simulink model "IEEE14_case"  (R2024b)
settings: Solver=FixedStepAuto  StartTime=0  StopTime=2  FixedStep=1e-7  RelTol=1e-3
values from neighbouring files (symbols this model uses):
  GFL_15_Bva = 0.009    [IEEE14_parameters.m]
  GFL_15_C_bus_pu = 7.179419    [IEEE14_parameters.m]
  GFL_15_f0 = 60    [IEEE14_parameters.m]
  GFL_15_I_id = 691.26967    [IEEE14_parameters.m]
  GFL_15_I_iq = 691.26967    [IEEE14_parameters.m]
  GFL_15_I_od = 45.2207    [IEEE14_parameters.m]
  GFL_15_I_oq = 45.2207    [IEEE14_parameters.m]
  GFL_15_I_pll = 0.78    [IEEE14_parameters.m]
  GFL_15_Kdi = 0.09    [IEEE14_parameters.m]
  GFL_15_Kdo = 0.9    [IEEE14_parameters.m]
  GFL_15_Kqi = 0.09    [IEEE14_parameters.m]
  GFL_15_Kqo = 0.9    [IEEE14_parameters.m]
  GFL_15_Lg_pu = 0.631447    [IEEE14_parameters.m]
  GFL_15_mode = 1    [IEEE14_parameters.m]
  GFL_15_P_id = 3.7166    [IEEE14_parameters.m]
  GFL_15_P_iq = 3.7166    [IEEE14_parameters.m]
  GFL_15_P_od = 0.4798    [IEEE14_parameters.m]
  GFL_15_P_oq = 0.4798    [IEEE14_parameters.m]
  GFL_15_P_pll = 290.42    [IEEE14_parameters.m]
  GFL_15_Qe_ref = 0.2    [IEEE14_parameters.m]
  GFL_15_Rg_pu = 0.024016    [IEEE14_parameters.m]
  GFL_15_Sbase = 1.000000e+4    (= 10000)    [IEEE14_parameters.m]
  GFL_15_Tdi = 0.01    [IEEE14_parameters.m]
  GFL_15_Tdo = 0.2    [IEEE14_parameters.m]
  GFL_15_Tqi = 0.01    [IEEE14_parameters.m]
  GFL_15_Tqo = 0.2    [IEEE14_parameters.m]
  GFL_15_Vbase = 380    [IEEE14_parameters.m]
  GFL_15_Vdc_ref = 1.011475    [IEEE14_parameters.m]
  GFL_15_Vdcbase = 700    [IEEE14_parameters.m]
  GFL_15_vq_ref = 0    [IEEE14_parameters.m]
  GFL_16_Bva = 0.002    [IEEE14_parameters.m]
  GFL_16_C_bus_pu = 7.179419    [IEEE14_parameters.m]
  GFL_16_f0 = 60    [IEEE14_parameters.m]
  GFL_16_I_id = 691.26967    [IEEE14_parameters.m]
  GFL_16_I_iq = 691.26967    [IEEE14_parameters.m]
  GFL_16_I_od = 45.2207    [IEEE14_parameters.m]
  GFL_16_I_oq = 45.2207    [IEEE14_parameters.m]
  GFL_16_I_pll = 0.78    [IEEE14_parameters.m]
  GFL_16_Kdi = 0.05    [IEEE14_parameters.m]
  GFL_16_Kdo = 0.5    [IEEE14_parameters.m]
  GFL_16_Kqi = 0.05    [IEEE14_parameters.m]
  GFL_16_Kqo = 0.5    [IEEE14_parameters.m]
  GFL_16_Lg_pu = 0.631447    [IEEE14_parameters.m]
  GFL_16_mode = 1    [IEEE14_parameters.m]
  GFL_16_P_id = 3.7166    [IEEE14_parameters.m]
  GFL_16_P_iq = 3.7166    [IEEE14_parameters.m]
  GFL_16_P_od = 0.4798    [IEEE14_parameters.m]
  GFL_16_P_oq = 0.4798    [IEEE14_parameters.m]
  GFL_16_P_pll = 290.42    [IEEE14_parameters.m]
  GFL_16_Qe_ref = 0.2    [IEEE14_parameters.m]
  GFL_16_Rg_pu = 0.024016    [IEEE14_parameters.m]
  GFL_16_Sbase = 1.000000e+4    (= 10000)    [IEEE14_parameters.m]
  GFL_16_Tdi = 0.01    [IEEE14_parameters.m]
  GFL_16_Tdo = 0.2    [IEEE14_parameters.m]
  GFL_16_Tqi = 0.01    [IEEE14_parameters.m]
  GFL_16_Tqo = 0.2    [IEEE14_parameters.m]
  GFL_16_Vbase = 380    [IEEE14_parameters.m]
  GFL_16_Vdc_ref = 1.01144    [IEEE14_parameters.m]
  GFL_16_Vdcbase = 700    [IEEE14_parameters.m]
  GFL_16_vq_ref = 0    [IEEE14_parameters.m]
  GFL_17_Bva = 0.002    [IEEE14_parameters.m]
  GFL_17_C_bus_pu = 7.179419    [IEEE14_parameters.m]
  GFL_17_f0 = 60    [IEEE14_parameters.m]
  GFL_17_I_id = 691.26967    [IEEE14_parameters.m]
  GFL_17_I_iq = 691.26967    [IEEE14_parameters.m]
  GFL_17_I_od = 45.2207    [IEEE14_parameters.m]
  GFL_17_I_oq = 45.2207    [IEEE14_parameters.m]
  GFL_17_I_pll = 0.78    [IEEE14_parameters.m]
  GFL_17_Kdi = 0.05    [IEEE14_parameters.m]
  GFL_17_Kdo = 0.5    [IEEE14_parameters.m]
  GFL_17_Kqi = 0.05    [IEEE14_parameters.m]
  GFL_17_Kqo = 0.5    [IEEE14_parameters.m]
  GFL_17_Lg_pu = 0.631447    [IEEE14_parameters.m]
  GFL_17_mode = 1    [IEEE14_parameters.m]
  GFL_17_P_id = 3.7166    [IEEE14_parameters.m]
  GFL_17_P_iq = 3.7166    [IEEE14_parameters.m]
  GFL_17_P_od = 0.4798    [IEEE14_parameters.m]
  GFL_17_P_oq = 0.4798    [IEEE14_parameters.m]
  GFL_17_P_pll = 290.42    [IEEE14_parameters.m]
  GFL_17_Qe_ref = 0.2    [IEEE14_parameters.m]
  GFL_17_Rg_pu = 0.024016    [IEEE14_parameters.m]
  GFL_17_Sbase = 1.000000e+4    (= 10000)    [IEEE14_parameters.m]
  GFL_17_Tdi = 0.01    [IEEE14_parameters.m]
  GFL_17_Tdo = 0.2    [IEEE14_parameters.m]
  GFL_17_Tqi = 0.01    [IEEE14_parameters.m]
  GFL_17_Tqo = 0.2    [IEEE14_parameters.m]
  GFL_17_Vbase = 380    [IEEE14_parameters.m]
  GFL_17_Vdc_ref = 1.011632    [IEEE14_parameters.m]
  GFL_17_Vdcbase = 700    [IEEE14_parameters.m]
  GFL_17_vq_ref = 0    [IEEE14_parameters.m]
  GFL_18_Bva = 0.002    [IEEE14_parameters.m]
  GFL_18_C_bus_pu = 7.179419    [IEEE14_parameters.m]
  GFL_18_f0 = 60    [IEEE14_parameters.m]
  GFL_18_I_id = 691.26967    [IEEE14_parameters.m]
  GFL_18_I_iq = 691.26967    [IEEE14_parameters.m]
  GFL_18_I_od = 45.2207    [IEEE14_parameters.m]
  GFL_18_I_oq = 45.2207    [IEEE14_parameters.m]
  GFL_18_I_pll = 0.78    [IEEE14_parameters.m]
  GFL_18_Kdi = 0.05    [IEEE14_parameters.m]
  GFL_18_Kdo = 0.5    [IEEE14_parameters.m]
  GFL_18_Kqi = 0.05    [IEEE14_parameters.m]
  GFL_18_Kqo = 0.5    [IEEE14_parameters.m]
  GFL_18_Lg_pu = 0.631447    [IEEE14_parameters.m]
  GFL_18_mode = 1    [IEEE14_parameters.m]
  GFL_18_P_id = 3.7166    [IEEE14_parameters.m]
  GFL_18_P_iq = 3.7166    [IEEE14_parameters.m]
  GFL_18_P_od = 0.4798    [IEEE14_parameters.m]
  GFL_18_P_oq = 0.4798    [IEEE14_parameters.m]
  GFL_18_P_pll = 290.42    [IEEE14_parameters.m]
  GFL_18_Qe_ref = 0.2    [IEEE14_parameters.m]
  GFL_18_Rg_pu = 0.024016    [IEEE14_parameters.m]
  GFL_18_Sbase = 1.000000e+4    (= 10000)    [IEEE14_parameters.m]
  GFL_18_Tdi = 0.01    [IEEE14_parameters.m]
  GFL_18_Tdo = 0.2    [IEEE14_parameters.m]
  GFL_18_Tqi = 0.01    [IEEE14_parameters.m]
  GFL_18_Tqo = 0.2    [IEEE14_parameters.m]
  GFL_18_Vbase = 380    [IEEE14_parameters.m]
  GFL_18_Vdc_ref = 1.011572    [IEEE14_parameters.m]
  GFL_18_Vdcbase = 700    [IEEE14_parameters.m]
  GFL_18_vq_ref = 0    [IEEE14_parameters.m]
  ... (+180 more)
(part 21 of 25)

== system IEEE14_case/SG_D_3/i_q_SG_D_3_block ==
  note: i_q_SG_D_3 in case14gfl
      | $-\frac{\sin\left(\theta _{\mathrm{SG},D,3}\right)\,\left(\psi _{q,\mathrm{SG},D,3}+\frac{\psi _{\mathrm{gq},\mathrm{SG},D,3}\,\left(x_{l}-x_{\mathrm{qdd}}\right)}{x_{l}-x_{\mathrm{qd}}}+\frac{\psi _{\mathrm{kq},\mathrm{SG},D,3}\,\left(x_{\mathrm{qd}}-x_{\mathrm{qdd}}\right)}{x_{l}-x_{\mathrm{qd}}}\right)}{x_{\mathrm{qdd}}}-\frac{\cos\left(\theta _{\mathrm{SG},D,3}\right)\,\left(\frac{\psi _{\mathrm{1d},\mathrm{SG},D,3}\,\left(x_{\mathrm{dd}}-x_{\mathrm{ddd}}\right)}{x_{\mathrm{dd}}-x_{l}}-\psi _{d,\mathrm{SG},D,3}+\frac{\psi _{\mathrm{fd},\mathrm{SG},D,3}\,\left(x_{\mathrm{ddd}}-x_{l}\right)}{x_{\mathrm{dd}}-x_{l}}\right)}{x_{\mathrm{ddd}}}$
      | Automatically generated on 2025-10-09 21:32:35 .
  State_psi_gq_SG_D_3_f7c17 : Inport
  State_psi_kq_SG_D_3_3c737 : Inport  Port=2
  State_psi_q_SG_D_3_2676a : Inport  Port=3
  State_theta_SG_D_3_9134c : Inport  Port=4
  State_psi_1d_SG_D_3_20d6e : Inport  Port=5
  State_psi_d_SG_D_3_ac680 : Inport  Port=6
  State_psi_fd_SG_D_3_bfdd7 : Inport  Port=7
  State_theta_SG_D_3_28037 : Inport  Port=8
  Add_4ac66 : Sum
  Add_5b661 : Sum
  Add_73f87 : Sum
  Add_78fd5 : Sum
  Add_d5f9a : Sum
  Add_dc007 : Sum
  Constant_-1_294ca : Constant  Value=-1
  Constant_-1_37339 : Constant  Value=-1
  Constant_-1_55310 : Constant  Value=-1
  Constant_-1_9bd92 : Constant  Value=-1
  Constant_-1_c0d20 : Constant  Value=-1
  Constant_x_dd_0e9f5 : Constant  Value=x_dd
  Constant_x_dd_107ff : Constant  Value=x_dd
  Constant_x_dd_c8724 : Constant  Value=x_dd
  Constant_x_ddd_0cb6a : Constant  Value=x_ddd
  Constant_x_ddd_61310 : Constant  Value=x_ddd
  Constant_x_ddd_6486c : Constant  Value=x_ddd
  Constant_x_l_1c7d3 : Constant  Value=x_l
  Constant_x_l_2af64 : Constant  Value=x_l
  Constant_x_l_57051 : Constant  Value=x_l
  Constant_x_l_7ebbc : Constant  Value=x_l
  Constant_x_l_96cf1 : Constant  Value=x_l
  Constant_x_l_9ef0a : Constant  Value=x_l
  Constant_x_qd_2bf67 : Constant  Value=x_qd
  Constant_x_qd_2ffe8 : Constant  Value=x_qd
  Constant_x_qd_baa51 : Constant  Value=x_qd
  Constant_x_qdd_09938 : Constant  Value=x_qdd
  Constant_x_qdd_17dfa : Constant  Value=x_qdd
  Constant_x_qdd_d3279 : Constant  Value=x_qdd
  Divide_0acbf : Product  Inputs=*/
  Divide_1822e : Product  Inputs=*/
  Divide_1e6a6 : Product  Inputs=*/
  Divide_3e273 : Product  Inputs=*/
  Divide_85360 : Product  Inputs=*/
  Divide_9dfff : Product  Inputs=*/
  MathFunc_cos_15d9a : Trigonometry  Operator=cos
  MathFunc_sin_902a4 : Trigonometry
  Product_0a2eb : Product
  Product_3ac28 : Product
  Product_4e1f4 : Product
  Product_5bceb : Product
  Product_723b0 : Product
  Product_7a0a1 : Product
  Product_9fc52 : Product
  Product_a5c0c : Product
  Product_ab665 : Product
  Product_b175d : Product
  Product_d7f70 : Product
  Subtract_0cd7d : Sum  Inputs=+-
  Subtract_369cd : Sum  Inputs=+-
  Subtract_41eed : Sum  Inputs=+-
  Subtract_9b04e : Sum  Inputs=+-
  Subtract_9e824 : Sum  Inputs=+-
  Subtract_b9947 : Sum  Inputs=+-
  Subtract_c0717 : Sum  Inputs=+-
  Blockout_i_q_SG_D_3_e7589 : Outport
  wires:
  Constant_x_qdd_09938/1 -> Divide_1e6a6/2
  Constant_x_dd_0e9f5/1 -> Subtract_b9947/1
  Constant_-1_37339/1 -> Product_3ac28/1
  Constant_-1_294ca/1 -> Product_b175d/1
  Constant_x_l_9ef0a/1 -> Product_b175d/2
  Subtract_41eed/1 -> Product_d7f70/1
  Constant_x_qdd_d3279/1 -> Subtract_c0717/2
  Constant_x_qdd_17dfa/1 -> Add_5b661/2
  Product_b175d/1 -> Add_5b661/1
  Constant_x_l_7ebbc/1 -> Subtract_b9947/2
  Add_d5f9a/1 -> Divide_9dfff/2
  Constant_x_l_57051/1 -> Product_3ac28/2
  Constant_x_ddd_61310/1 -> Subtract_369cd/1
  Constant_x_qd_2ffe8/1 -> Subtract_c0717/1
  Constant_-1_c0d20/1 -> Product_7a0a1/1
  Product_9fc52/1 -> Product_5bceb/1
  Constant_x_l_2af64/1 -> Product_7a0a1/2
  Product_5bceb/1 -> Divide_1822e/1
  State_psi_gq_SG_D_3_f7c17/1 -> Product_0a2eb/1
  Add_5b661/1 -> Product_0a2eb/2
  Subtract_b9947/1 -> Divide_1822e/2
  Product_3ac28/1 -> Add_d5f9a/1
  Divide_3e273/1 -> Add_4ac66/2
  Constant_x_qd_2bf67/1 -> Add_d5f9a/2
  State_psi_fd_SG_D_3_bfdd7/1 -> Product_4e1f4/1
  State_psi_kq_SG_D_3_3c737/1 -> Product_ab665/1
  Subtract_369cd/1 -> Product_4e1f4/2
  Subtract_c0717/1 -> Product_ab665/2
  Product_7a0a1/1 -> Add_73f87/1
  Constant_x_qd_baa51/1 -> Add_73f87/2
  Constant_x_l_96cf1/1 -> Subtract_369cd/2
  Constant_-1_55310/1 -> Product_9fc52/1
  State_psi_1d_SG_D_3_20d6e/1 -> Product_9fc52/2
  Constant_x_dd_c8724/1 -> Subtract_9b04e/1
  Constant_-1_9bd92/1 -> Product_723b0/1
  Constant_x_ddd_0cb6a/1 -> Subtract_9b04e/2
  Add_dc007/1 -> Product_723b0/2
  Product_0a2eb/1 -> Divide_9dfff/1
  Product_4e1f4/1 -> Divide_85360/1
  Product_ab665/1 -> Divide_0acbf/1
  Subtract_0cd7d/1 -> Divide_85360/2
  Add_73f87/1 -> Divide_0acbf/2
  Constant_x_ddd_6486c/1 -> Divide_3e273/2
  Subtract_9b04e/1 -> Product_5bceb/2
  Divide_9dfff/1 -> Subtract_9e824/1
  Divide_85360/1 -> Subtract_41eed/2
  Divide_0acbf/1 -> Subtract_9e824/2
  Constant_x_dd_107ff/1 -> Subtract_0cd7d/1
  Constant_x_l_1c7d3/1 -> Subtract_0cd7d/2
  Subtract_9e824/1 -> Add_dc007/1
  State_psi_q_SG_D_3_2676a/1 -> Add_dc007/2
  Divide_1822e/1 -> Add_78fd5/1
  MathFunc_sin_902a4/1 -> Product_a5c0c/2
  Product_723b0/1 -> Product_a5c0c/1
  State_psi_d_SG_D_3_ac680/1 -> Add_78fd5/2
  State_theta_SG_D_3_9134c/1 -> MathFunc_sin_902a4/1
  Add_78fd5/1 -> Subtract_41eed/1
  State_theta_SG_D_3_28037/1 -> MathFunc_cos_15d9a/1
  MathFunc_cos_15d9a/1 -> Product_d7f70/2
  Divide_1e6a6/1 -> Add_4ac66/1
  Product_a5c0c/1 -> Divide_1e6a6/1
  Product_d7f70/1 -> Divide_3e273/1
  Add_4ac66/1 -> Blockout_i_q_SG_D_3_e7589/1

== system IEEE14_case/SG_D_3/theta_SG_D_3_out_block ==
  note: theta_SG_D_3_out in case14gfl
      | $\theta _{\mathrm{SG},D,3}$
      | Automatically generated on 2025-10-09 21:32:40 .
  State_theta_SG_D_3_9fa07 : Inport
  Blockout_theta_SG_D_3_out_2c966 : Outport
  wires:
  State_theta_SG_D_3_9fa07/1 -> Blockout_theta_SG_D_3_out_2c966/1

== system IEEE14_case/SG_D_3/w_SG_D_3_out_block ==
  note: w_SG_D_3_out in case14gfl
      | $w_{\mathrm{SG},D,3}$
      | Automatically generated on 2025-10-09 21:32:39 .
  State_w_SG_D_3_f6ed4 : Inport
  Blockout_w_SG_D_3_out_ef88e : Outport
  wires:
  State_w_SG_D_3_f6ed4/1 -> Blockout_w_SG_D_3_out_ef88e/1

== system IEEE14_case/SG_D_6/T_e_SG_D_6_block ==
  note: T_e_SG_D_6 in case14gfl
      | $-\frac{\psi _{d,\mathrm{SG},D,6}\,\left(\psi _{q,\mathrm{SG},D,6}+\frac{\psi _{\mathrm{gq},\mathrm{SG},D,6}\,\left(x_{l}-x_{\mathrm{qdd}}\right)}{x_{l}-x_{\mathrm{qd}}}+\frac{\psi _{\mathrm{kq},\mathrm{SG},D,6}\,\left(x_{\mathrm{qd}}-x_{\mathrm{qdd}}\right)}{x_{l}-x_{\mathrm{qd}}}\right)}{x_{\mathrm{qdd}}}-\frac{\psi _{q,\mathrm{SG},D,6}\,\left(\frac{\psi _{\mathrm{1d},\mathrm{SG},D,6}\,\left(x_{\mathrm{dd}}-x_{\mathrm{ddd}}\right)}{x_{\mathrm{dd}}-x_{l}}-\psi _{d,\mathrm{SG},D,6}+\frac{\psi _{\mathrm{fd},\mathrm{SG},D,6}\,\left(x_{\mathrm{ddd}}-x_{l}\right)}{x_{\mathrm{dd}}-x_{l}}\right)}{x_{\mathrm{ddd}}}$
      | Automatically generated on 2025-10-09 21:33:40 .
  State_psi_d_SG_D_6_50e5d : Inport
  State_psi_gq_SG_D_6_6e720 : Inport  Port=2
  State_psi_kq_SG_D_6_3291f : Inport  Port=3
  State_psi_q_SG_D_6_ac522 : Inport  Port=4
  State_psi_q_SG_D_6_09a29 : Inport  Port=5
  State_psi_1d_SG_D_6_60340 : Inport  Port=6
  State_psi_d_SG_D_6_bc7a5 : Inport  Port=7
  State_psi_fd_SG_D_6_b7b2b : Inport  Port=8
  Add_07e22 : Sum
  Add_8c5ef : Sum
  Add_a9dc7 : Sum
  Add_ba390 : Sum
  Add_eb995 : Sum
  Add_f4f44 : Sum
  Constant_-1_18776 : Constant  Value=-1
  Constant_-1_1eab1 : Constant  Value=-1
  Constant_-1_8eb32 : Constant  Value=-1
  Constant_-1_bd0bf : Constant  Value=-1
  Constant_-1_f585a : Constant  Value=-1
  Constant_x_dd_3f9f6 : Constant  Value=x_dd
  Constant_x_dd_921da : Constant  Value=x_dd
  Constant_x_dd_bb25b : Constant  Value=x_dd
  Constant_x_ddd_2201b : Constant  Value=x_ddd
  Constant_x_ddd_42d4a : Constant  Value=x_ddd
  Constant_x_ddd_a1cba : Constant  Value=x_ddd
  Constant_x_l_61e5d : Constant  Value=x_l
  Constant_x_l_8bb7b : Constant  Value=x_l
  Constant_x_l_9966c : Constant  Value=x_l
  Constant_x_l_b6875 : Constant  Value=x_l
  Constant_x_l_c9181 : Constant  Value=x_l
  Constant_x_l_efaf6 : Constant  Value=x_l
  Constant_x_qd_59b3c : Constant  Value=x_qd
  Constant_x_qd_611d3 : Constant  Value=x_qd
  Constant_x_qd_b9d48 : Constant  Value=x_qd
  Constant_x_qdd_11045 : Constant  Value=x_qdd
  Constant_x_qdd_37290 : Constant  Value=x_qdd
  Constant_x_qdd_e46cf : Constant  Value=x_qdd
  Divide_0725c : Product  Inputs=*/
  Divide_23c16 : Product  Inputs=*/
  Divide_33909 : Product  Inputs=*/
  Divide_4ca5c : Product  Inputs=*/
  Divide_4e2d7 : Product  Inputs=*/
  Divide_f7d6a : Product  Inputs=*/
  Product_0edde : Product
  Product_1c9b7 : Product
  Product_2ebb8 : Product
  Product_4df84 : Product
  Product_69977 : Product
  Product_7bc7e : Product
  Product_a39ae : Product
  Product_d7bc6 : Product
  Product_de235 : Product
  Product_eeb4e : Product
  Product_f572e : Product
  Subtract_3ce0b : Sum  Inputs=+-
  Subtract_65510 : Sum  Inputs=+-
  Subtract_6ad1d : Sum  Inputs=+-
  Subtract_7e2a6 : Sum  Inputs=+-
  Subtract_adf61 : Sum  Inputs=+-
  Subtract_d3337 : Sum  Inputs=+-
  Subtract_e7903 : Sum  Inputs=+-
  Blockout_T_e_SG_D_6_1c5ce : Outport
  wires:
  Constant_x_ddd_a1cba/1 -> Divide_f7d6a/2
  Constant_-1_f585a/1 -> Product_69977/1
  Constant_x_qd_59b3c/1 -> Add_07e22/2
  Constant_-1_18776/1 -> Product_0edde/1
  Add_07e22/1 -> Divide_4ca5c/2
  Constant_x_l_c9181/1 -> Product_0edde/2
  Constant_-1_1eab1/1 -> Product_d7bc6/1
  Product_0edde/1 -> Add_ba390/1
  Constant_x_qdd_37290/1 -> Subtract_7e2a6/2
  Add_eb995/1 -> Product_1c9b7/2
  Subtract_6ad1d/1 -> Product_a39ae/2
  Constant_x_ddd_42d4a/1 -> Subtract_6ad1d/1
  Constant_x_qdd_e46cf/1 -> Add_ba390/2
  Constant_-1_bd0bf/1 -> Product_7bc7e/1
  Constant_x_qd_611d3/1 -> Subtract_7e2a6/1
  Subtract_65510/1 -> Product_de235/2
  Constant_x_dd_921da/1 -> Subtract_65510/1
  Constant_x_l_61e5d/1 -> Product_69977/2
  Product_1c9b7/1 -> Divide_4e2d7/1
  Constant_-1_8eb32/1 -> Product_2ebb8/1
  Constant_x_l_efaf6/1 -> Product_2ebb8/2
  Add_f4f44/1 -> Blockout_T_e_SG_D_6_1c5ce/1
  State_psi_1d_SG_D_6_60340/1 -> Product_d7bc6/2
  Constant_x_ddd_2201b/1 -> Subtract_65510/2
  State_psi_gq_SG_D_6_6e720/1 -> Product_f572e/1
  Add_ba390/1 -> Product_f572e/2
  Product_69977/1 -> Add_07e22/1
  State_psi_kq_SG_D_6_3291f/1 -> Product_4df84/1
  Subtract_7e2a6/1 -> Product_4df84/2
  Product_2ebb8/1 -> Add_8c5ef/1
  Constant_x_qd_b9d48/1 -> Add_8c5ef/2
  Product_d7bc6/1 -> Product_de235/1
  Subtract_3ce0b/1 -> Divide_23c16/2
  Add_8c5ef/1 -> Divide_0725c/2
  Constant_x_dd_bb25b/1 -> Subtract_3ce0b/1
  Constant_x_l_9966c/1 -> Subtract_3ce0b/2
  Constant_x_l_8bb7b/1 -> Subtract_6ad1d/2
  Subtract_e7903/1 -> Add_eb995/1
  Product_f572e/1 -> Divide_4ca5c/1
  Subtract_d3337/1 -> Divide_33909/2
  Constant_x_dd_3f9f6/1 -> Subtract_d3337/1
  Product_4df84/1 -> Divide_0725c/1
  Product_de235/1 -> Divide_23c16/1
  State_psi_d_SG_D_6_50e5d/1 -> Product_7bc7e/2
  Product_a39ae/1 -> Divide_33909/1
  State_psi_fd_SG_D_6_b7b2b/1 -> Product_a39ae/1
  Divide_4e2d7/1 -> Add_f4f44/1
  Constant_x_l_b6875/1 -> Subtract_d3337/2
  Divide_4ca5c/1 -> Subtract_e7903/1
  Divide_33909/1 -> Subtract_adf61/2
  Divide_0725c/1 -> Subtract_e7903/2
  Divide_23c16/1 -> Add_a9dc7/1
  State_psi_d_SG_D_6_bc7a5/1 -> Add_a9dc7/2
  State_psi_q_SG_D_6_ac522/1 -> Add_eb995/2
  Add_a9dc7/1 -> Subtract_adf61/1
  Product_eeb4e/1 -> Divide_f7d6a/1
  Product_7bc7e/1 -> Product_1c9b7/1
  State_psi_q_SG_D_6_09a29/1 -> Product_eeb4e/1
  Subtract_adf61/1 -> Product_eeb4e/2
  Constant_x_qdd_11045/1 -> Divide_4e2d7/2
  Divide_f7d6a/1 -> Add_f4f44/2

== system IEEE14_case/SG_D_6/d_E_fd_SG_D_6_block ==
  note: d_E_fd_SG_D_6 in case14gfl
      | $\frac{V_{f,\mathrm{SG},D,6}-E_{\mathrm{fd},\mathrm{SG},D,6}\,K_{E}}{T_{E}}$
      | Automatically generated on 2025-10-09 21:33:25 .
  State_E_fd_SG_D_6_93beb : Inport
  State_V_f_SG_D_6_97849 : Inport  Port=2
  Add_07863 : Sum
  Constant_-1_1bdcc : Constant  Value=-1
  Constant_K_E_feb12 : Constant  Value=K_E
  Constant_T_E_5779f : Constant  Value=T_E
  Divide_1f966 : Product  Inputs=*/
  Product_92caf : Product
  Product_d9fed : Product
  Blockout_d_E_fd_SG_D_6_64fbc : Outport
  wires:
  State_V_f_SG_D_6_97849/1 -> Add_07863/2
  State_E_fd_SG_D_6_93beb/1 -> Product_d9fed/2
  Constant_-1_1bdcc/1 -> Product_d9fed/1
  Product_d9fed/1 -> Product_92caf/1
  Constant_K_E_feb12/1 -> Product_92caf/2
  Add_07863/1 -> Divide_1f966/1
  Divide_1f966/1 -> Blockout_d_E_fd_SG_D_6_64fbc/1
  Product_92caf/1 -> Add_07863/1
  Constant_T_E_5779f/1 -> Divide_1f966/2

== system IEEE14_case/SG_D_6/d_Px_1_SG_D_6_block ==
  note: d_Px_1_SG_D_6 in case14gfl
      | $\frac{w_{\mathrm{SG},D,6}-2\,\pi \,f_{0}}{T_{w}}-\frac{\mathrm{Px}_{1,\mathrm{SG},D,6}}{T_{w}}$
      | Automatically generated on 2025-10-09 21:33:26 .
  State_Px_1_SG_D_6_18725 : Inport
  State_w_SG_D_6_e1d55 : Inport  Port=2
  Add_0fab3 : Sum
  Add_bc308 : Sum
  Constant_-1_2e521 : Constant  Value=-1
  Constant_-2.0_2d352 : Constant  Value=-2.0
  Constant_T_w_15733 : Constant  Value=T_w
  Constant_T_w_25c4d : Constant  Value=T_w
  Constant_f0_a2ec4 : Constant  Value=f0
  Constant_pi_58c78 : Constant  Value=pi
  Divide_2ed8f : Product  Inputs=*/
  Divide_9e884 : Product  Inputs=*/
  Product_7c40c : Product
  Product_d036b : Product
  Product_e52e7 : Product
  Blockout_d_Px_1_SG_D_6_40901 : Outport
  wires:
  Constant_-2.0_2d352/1 -> Product_7c40c/1
  Product_e52e7/1 -> Add_0fab3/1
  Constant_pi_58c78/1 -> Product_7c40c/2
  Constant_f0_a2ec4/1 -> Product_e52e7/2
  Product_7c40c/1 -> Product_e52e7/1
  Constant_-1_2e521/1 -> Product_d036b/1
  State_w_SG_D_6_e1d55/1 -> Add_0fab3/2
  State_Px_1_SG_D_6_18725/1 -> Product_d036b/2
  Product_d036b/1 -> Divide_9e884/1
  Constant_T_w_15733/1 -> Divide_9e884/2
  Add_0fab3/1 -> Divide_2ed8f/1
  Constant_T_w_25c4d/1 -> Divide_2ed8f/2
  Divide_9e884/1 -> Add_bc308/1
  Divide_2ed8f/1 -> Add_bc308/2
  Add_bc308/1 -> Blockout_d_Px_1_SG_D_6_40901/1

== system IEEE14_case/SG_D_6/d_Px_2_SG_D_6_block ==
  note: d_Px_2_SG_D_6 in case14gfl
      | $\frac{\mathrm{Px}_{1,\mathrm{SG},D,6}-T_{2}\,\left(\frac{\mathrm{Px}_{1,\mathrm{SG},D,6}}{T_{w}}-\frac{w_{\mathrm{SG},D,6}-2\,\pi \,f_{0}}{T_{w}}\right)}{T_{1}}-\frac{\mathrm{Px}_{2,\mathrm{SG},D,6}}{T_{1}}$
      | Automatically generated on 2025-10-09 21:33:27 .
  State_Px_2_SG_D_6_5cdcf : Inport
  State_Px_1_SG_D_6_26ff3 : Inport  Port=2
  State_Px_1_SG_D_6_357af : Inport  Port=3
  State_w_SG_D_6_5d512 : Inport  Port=4
  Add_242fa : Sum
  Add_543fb : Sum
  Add_9bc8c : Sum
  Add_cd322 : Sum
  Constant_-1_2147e : Constant  Value=-1
  Constant_-1_e132c : Constant  Value=-1
  Constant_-2.0_babc7 : Constant  Value=-2.0
  Constant_T_1_bb663 : Constant  Value=T_1
  Constant_T_1_c4036 : Constant  Value=T_1
  Constant_T_2_2f3fa : Constant  Value=T_2
  Constant_T_w_24d18 : Constant  Value=T_w
  Constant_T_w_8bff3 : Constant  Value=T_w
  Constant_f0_0491e : Constant  Value=f0
  Constant_pi_f9abd : Constant  Value=pi
  Divide_1712f : Product  Inputs=*/
  Divide_6dcdf : Product  Inputs=*/
  Divide_9ba3d : Product  Inputs=*/
  Divide_acd1d : Product  Inputs=*/
  Product_1e677 : Product
  Product_27f1c : Product
  Product_50e25 : Product
  Product_7af97 : Product
  Product_7e1a3 : Product
  Blockout_d_Px_2_SG_D_6_3663f : Outport
  wires:
  Constant_-2.0_babc7/1 -> Product_50e25/1
  Product_1e677/1 -> Add_9bc8c/1
  Constant_pi_f9abd/1 -> Product_50e25/2
  State_Px_1_SG_D_6_357af/1 -> Product_27f1c/2
  Constant_f0_0491e/1 -> Product_1e677/2
  Constant_T_1_bb663/1 -> Divide_6dcdf/2
  Product_50e25/1 -> Product_1e677/1
  Constant_-1_e132c/1 -> Product_27f1c/1
  State_w_SG_D_6_5d512/1 -> Add_9bc8c/2
  Product_27f1c/1 -> Divide_acd1d/1
  Constant_T_w_8bff3/1 -> Divide_acd1d/2
  Add_9bc8c/1 -> Divide_1712f/1
  Constant_T_w_24d18/1 -> Divide_1712f/2
  Divide_acd1d/1 -> Add_cd322/1
  Divide_1712f/1 -> Add_cd322/2
  State_Px_2_SG_D_6_5cdcf/1 -> Product_7af97/2
  Constant_T_2_2f3fa/1 -> Product_7e1a3/1
  Add_cd322/1 -> Product_7e1a3/2
  Constant_-1_2147e/1 -> Product_7af97/1
  State_Px_1_SG_D_6_26ff3/1 -> Add_242fa/1
  Product_7e1a3/1 -> Add_242fa/2
  Product_7af97/1 -> Divide_9ba3d/1
  Add_543fb/1 -> Blockout_d_Px_2_SG_D_6_3663f/1
  Constant_T_1_c4036/1 -> Divide_9ba3d/2
  Add_242fa/1 -> Divide_6dcdf/1
  Divide_9ba3d/1 -> Add_543fb/1
  Divide_6dcdf/1 -> Add_543fb/2

== system IEEE14_case/SG_D_6/d_Px_3_SG_D_6_block ==
  note: d_Px_3_SG_D_6 in case14gfl
      | $\frac{\mathrm{Px}_{2,\mathrm{SG},D,6}+T_{4}\,\left(\frac{\mathrm{Px}_{1,\mathrm{SG},D,6}-T_{2}\,\left(\frac{\mathrm{Px}_{1,\mathrm{SG},D,6}}{T_{w}}-\frac{w_{\mathrm{SG},D,6}-2\,\pi \,f_{0}}{T_{w}}\right)}{T_{1}}-\frac{\mathrm{Px}_{2,\mathrm{SG},D,6}}{T_{1}}\right)}{T_{3}}-\frac{\mathrm{Px}_{3,\mathrm{SG},D,6}}{T_{3}}$
      | Automatically generated on 2025-10-09 21:33:29 .
  State_Px_3_SG_D_6_9df2d : Inport
  State_Px_2_SG_D_6_2857b : Inport  Port=2
  State_Px_2_SG_D_6_eb0dd : Inport  Port=3
  State_Px_1_SG_D_6_c3a44 : Inport  Port=4
  State_Px_1_SG_D_6_b27f4 : Inport  Port=5
  State_w_SG_D_6_5f02d : Inport  Port=6
  Add_1e205 : Sum
  Add_5dbc7 : Sum
  Add_a8038 : Sum
  Add_c210d : Sum
  Add_cadc6 : Sum
  Add_f15ac : Sum
  Constant_-1_5809a : Constant  Value=-1
  Constant_-1_66981 : Constant  Value=-1
  Constant_-1_83692 : Constant  Value=-1
  Constant_-2.0_fcf47 : Constant  Value=-2.0
  Constant_T_1_20858 : Constant  Value=T_1
  Constant_T_1_a342f : Constant  Value=T_1
  Constant_T_2_d497b : Constant  Value=T_2
  Constant_T_3_36427 : Constant  Value=T_3
  Constant_T_3_a4b23 : Constant  Value=T_3
  Constant_T_4_33fd0 : Constant  Value=T_4
  Constant_T_w_863c7 : Constant  Value=T_w
  Constant_T_w_8faca : Constant  Value=T_w
  Constant_f0_39412 : Constant  Value=f0
  Constant_pi_db662 : Constant  Value=pi
  Divide_0d6f9 : Product  Inputs=*/
  Divide_18fa6 : Product  Inputs=*/
  Divide_3de34 : Product  Inputs=*/
  Divide_a01f5 : Product  Inputs=*/
  Divide_f0387 : Product  Inputs=*/
  Divide_f0c68 : Product  Inputs=*/
  Product_00e30 : Product
  Product_2da59 : Product
  Product_6e57d : Product
  Product_c4fce : Product
  Product_cbbcd : Product
  Product_d1479 : Product
  Product_d63f7 : Product
  Blockout_d_Px_3_SG_D_6_17e90 : Outport
  wires:
  Constant_-2.0_fcf47/1 -> Product_2da59/1
  Add_1e205/1 -> Blockout_d_Px_3_SG_D_6_17e90/1
  Product_6e57d/1 -> Add_cadc6/1
  Add_c210d/1 -> Divide_3de34/1
  Constant_pi_db662/1 -> Product_2da59/2
  State_Px_1_SG_D_6_b27f4/1 -> Product_d1479/2
  Constant_f0_39412/1 -> Product_6e57d/2
  Product_2da59/1 -> Product_6e57d/1
  Constant_T_w_863c7/1 -> Divide_a01f5/2
  Constant_-1_66981/1 -> Product_d1479/1
  State_w_SG_D_6_5f02d/1 -> Add_cadc6/2
  Product_d1479/1 -> Divide_a01f5/1
  Add_cadc6/1 -> Divide_18fa6/1
  Constant_-1_83692/1 -> Product_c4fce/1
  Constant_T_w_8faca/1 -> Divide_18fa6/2
  Divide_a01f5/1 -> Add_a8038/1
  Divide_18fa6/1 -> Add_a8038/2
  Constant_T_3_36427/1 -> Divide_f0387/2
  Constant_T_2_d497b/1 -> Product_cbbcd/1
  Add_a8038/1 -> Product_cbbcd/2
  State_Px_2_SG_D_6_eb0dd/1 -> Product_c4fce/2
  State_Px_1_SG_D_6_c3a44/1 -> Add_c210d/1
  Product_cbbcd/1 -> Add_c210d/2
  Constant_T_3_a4b23/1 -> Divide_0d6f9/2
  Product_c4fce/1 -> Divide_f0c68/1
  Constant_T_1_a342f/1 -> Divide_f0c68/2
  Constant_T_1_20858/1 -> Divide_3de34/2
  Divide_f0c68/1 -> Add_5dbc7/1
  Divide_3de34/1 -> Add_5dbc7/2
  Constant_T_4_33fd0/1 -> Product_00e30/1
  Add_5dbc7/1 -> Product_00e30/2
  Divide_0d6f9/1 -> Add_1e205/2
  Constant_-1_5809a/1 -> Product_d63f7/1
  State_Px_3_SG_D_6_9df2d/1 -> Product_d63f7/2
  State_Px_2_SG_D_6_2857b/1 -> Add_f15ac/1
  Product_00e30/1 -> Add_f15ac/2
  Product_d63f7/1 -> Divide_f0387/1
  Add_f15ac/1 -> Divide_0d6f9/1
  Divide_f0387/1 -> Add_1e205/1

== system IEEE14_case/SG_D_6/d_R_f_SG_D_6_block ==
  note: d_R_f_SG_D_6 in case14gfl
      | $-\frac{R_{f,\mathrm{SG},D,6}-\frac{E_{\mathrm{fd},\mathrm{SG},D,6}\,K_{F}}{T_{F}}}{T_{F}}$
      | Automatically generated on 2025-10-09 21:33:24 .
  State_E_fd_SG_D_6_ceac9 : Inport
  State_R_f_SG_D_6_39afc : Inport  Port=2
  Constant_K_F_5195d : Constant  Value=K_F
  Constant_T_F_9963a : Constant  Value=T_F
  Constant_T_F_ad259 : Constant  Value=T_F
  Divide_b6cd7 : Product  Inputs=*/
  Divide_b7acf : Product  Inputs=*/
  Product_d1215 : Product
  Subtract_9e141 : Sum  Inputs=+-
  Blockout_d_R_f_SG_D_6_b769e : Outport
  wires:
  State_E_fd_SG_D_6_ceac9/1 -> Product_d1215/1
  Constant_K_F_5195d/1 -> Product_d1215/2
  Product_d1215/1 -> Divide_b6cd7/1
  Divide_b6cd7/1 -> Subtract_9e141/1
  Constant_T_F_9963a/1 -> Divide_b7acf/2
  Constant_T_F_ad259/1 -> Divide_b6cd7/2
  State_R_f_SG_D_6_39afc/1 -> Subtract_9e141/2
  Subtract_9e141/1 -> Divide_b7acf/1
  Divide_b7acf/1 -> Blockout_d_R_f_SG_D_6_b769e/1

== system IEEE14_case/SG_D_6/d_T_m_SG_D_6_block ==
  note: d_T_m_SG_D_6 in case14gfl
      | $-\frac{T_{m,\mathrm{SG},D,6}-T_{0}+\frac{\mathrm{SpeedPara}\,\left(w_{\mathrm{SG},D,6}-w_{\mathrm{ref}}\right)}{2\,f_{0}\,\pi }}{T_{\mathrm{speed}}}$
      | Automatically generated on 2025-10-09 21:33:16 .
  State_w_SG_D_6_e6164 : Inport
  State_T_m_SG_D_6_02315 : Inport  Port=2
  Add_0f60a : Sum
  Add_82741 : Sum
  Constant_-1_eccf6 : Constant  Value=-1
  Constant_2.0_92ac1 : Constant  Value=2.0
  Constant_SpeedPara_d6c6f : Constant  Value=SpeedPara
  Constant_T_0_c469d : Constant  Value=T_0
  Constant_T_speed_0c5b3 : Constant  Value=T_speed
  Constant_f0_9f40f : Constant  Value=f0
  Constant_pi_7d0a9 : Constant  Value=pi
  Constant_w_ref_d0a96 : Constant  Value=w_ref
  Divide_4cfe9 : Product  Inputs=*/
  Divide_6312a : Product  Inputs=*/
  Product_519a5 : Product
  Product_63b0c : Product
  Product_7ad8e : Product
  Product_aaaee : Product
  Subtract_24a76 : Sum  Inputs=+-
  Blockout_d_T_m_SG_D_6_83af8 : Outport
  wires:
  Constant_-1_eccf6/1 -> Product_aaaee/1
  Constant_w_ref_d0a96/1 -> Add_0f60a/2
  State_w_SG_D_6_e6164/1 -> Product_aaaee/2
  Product_aaaee/1 -> Add_0f60a/1
  Constant_2.0_92ac1/1 -> Product_7ad8e/1
  Constant_pi_7d0a9/1 -> Product_7ad8e/2
  Add_0f60a/1 -> Product_63b0c/2
  Constant_SpeedPara_d6c6f/1 -> Product_63b0c/1
  Product_7ad8e/1 -> Product_519a5/1
  Constant_f0_9f40f/1 -> Product_519a5/2
  Product_63b0c/1 -> Divide_6312a/1
  Add_82741/1 -> Subtract_24a76/1
  Product_519a5/1 -> Divide_6312a/2
  Divide_6312a/1 -> Add_82741/1
  Constant_T_0_c469d/1 -> Add_82741/2
  State_T_m_SG_D_6_02315/1 -> Subtract_24a76/2
  Subtract_24a76/1 -> Divide_4cfe9/1
  Constant_T_speed_0c5b3/1 -> Divide_4cfe9/2
  Divide_4cfe9/1 -> Blockout_d_T_m_SG_D_6_83af8/1

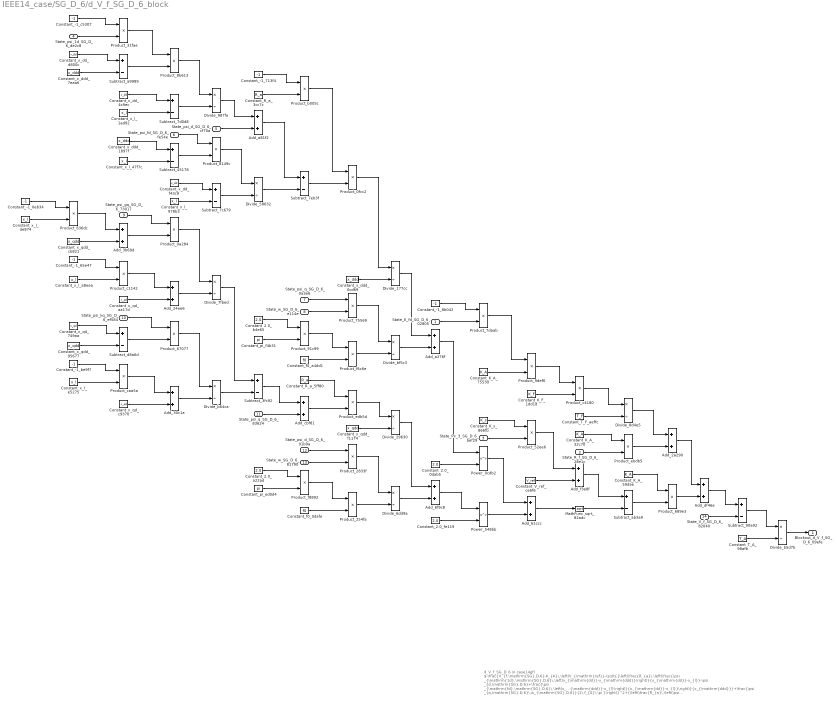
== system IEEE14_case/SG_D_6/d_V_f_SG_D_6_block ==
  note: d_V_f_SG_D_6 in case14gfl
      | $-\frac{V_{f,\mathrm{SG},D,6}-K_{A}\,\left(V_{\mathrm{ref}}-\sqrt{{\left(\frac{R_{a}\,\left(\frac{\psi _{\mathrm{1d},\mathrm{SG},D,6}\,\left(x_{\mathrm{dd}}-x_{\mathrm{ddd}}\right)}{x_{\mathrm{dd}}-x_{l}}-\psi _{d,\mathrm{SG},D,6}+\frac{\psi _{\mathrm{fd},\mathrm{SG},D,6}\,\left(x_{\mathrm{ddd}}-x_{l}\right)}{x_{\mathrm{dd}}-x_{l}}\right)}{x_{\mathrm{ddd}}}+\frac{\psi _{q,\mathrm{SG},D,6}\,w_{\mathrm{SG},D,6}}{2\,f_{0}\,\pi }\right)}^2+{\left(\frac{R_{a}\,\left(\psi _{q,\mathrm{SG},D,6}+\frac{\psi _{\mathrm{gq},\mathrm{SG},D,6}\,\left(x_{l}-x_{\mathrm{qdd}}\right)}{x_{l}-x_{\mathrm{qd}}}+\frac{\psi _{\mathrm{kq},\mathrm{SG},D,6}\,\left(x_{\mathrm{qd}}-x_{\mathrm{qdd}}\right)}{x_{l}-x_{\mathrm{qd}}}\right)}{x_{\mathrm{qdd}}}+\frac{\psi _{d,\mathrm{SG},D,6}\,w_{\mathrm{SG},D,6}}{2\,f_{0}\,\pi }\right)}^2}+K_{s}\,\mathrm{Px}_{3,\mathrm{SG},D,6}\right)-K_{A}\,R_{f,\mathrm{SG},D,6}+\frac{E_{\mathrm{fd},\mathrm{SG},D,6}\,K_{A}\,K_{F}}{T_{F}}}{T_{A}}$
      | Automatically generated on 2025-10-09 21:33:23 .
  State_E_fd_SG_D_6_02805 : Inport
  State_R_f_SG_D_6_28e1c : Inport  Port=2
  State_Px_3_SG_D_6_bef29 : Inport  Port=3
  State_psi_1d_SG_D_6_de2c8 : Inport  Port=4
  State_psi_d_SG_D_6_cf70a : Inport  Port=5
  State_psi_fd_SG_D_6_fe54e : Inport  Port=6
  State_psi_q_SG_D_6_0a3e6 : Inport  Port=7
  State_w_SG_D_6_e114e : Inport  Port=8
  State_psi_gq_SG_D_6_73017 : Inport  Port=9
  State_psi_kq_SG_D_6_ef584 : Inport  Port=10
  State_psi_q_SG_D_6_83624 : Inport  Port=11
  State_psi_d_SG_D_6_91b9a : Inport  Port=12
  State_w_SG_D_6_81790 : Inport  Port=13
  State_V_f_SG_D_6_82040 : Inport  Port=14
  Add_24ee6 : Sum
  Add_2a290 : Sum
  Add_30c1a : Sum
  Add_3b69d : Sum
  Add_61ccc : Sum
  Add_6f9c8 : Sum
  Add_a276f : Sum
  Add_a81f2 : Sum
  Add_cbf81 : Sum
  Add_df46e : Sum
  Add_f3e8f : Sum
  Constant_-1_0eb34 : Constant  Value=-1
  Constant_-1_65e47 : Constant  Value=-1
  Constant_-1_713f4 : Constant  Value=-1
  Constant_-1_8b042 : Constant  Value=-1
  Constant_-1_be9f7 : Constant  Value=-1
  Constant_-1_c5307 : Constant  Value=-1
  Constant_2.0_0dab5 : Constant  Value=2.0
  Constant_2.0_a22ad : Constant  Value=2.0
  Constant_2.0_b4e65 : Constant  Value=2.0
  Constant_2.0_fe119 : Constant  Value=2.0
  Constant_K_A_32c70 : Constant  Value=K_A
  Constant_K_A_59dae : Constant  Value=K_A
  Constant_K_A_7553d : Constant  Value=K_A
  Constant_K_F_1dd1d : Constant  Value=K_F
  Constant_K_s_866fb : Constant  Value=K_s
  Constant_R_a_3cc7c : Constant  Value=R_a
  Constant_R_a_5ff80 : Constant  Value=R_a
  Constant_T_A_98afb : Constant  Value=T_A
  Constant_T_F_aeffc : Constant  Value=T_F
  Constant_V_ref_ce6f6 : Constant  Value=V_ref
  Constant_f0_0dafe : Constant  Value=f0
  Constant_f0_a4dd1 : Constant  Value=f0
  Constant_pi_ed0d4 : Constant  Value=pi
  Constant_pi_f4b31 : Constant  Value=pi
  Constant_x_dd_4c9ec : Constant  Value=x_dd
  Constant_x_dd_d800c : Constant  Value=x_dd
  Constant_x_dd_f43c9 : Constant  Value=x_dd
  Constant_x_ddd_0cd69 : Constant  Value=x_ddd
  Constant_x_ddd_1897f : Constant  Value=x_ddd
  Constant_x_ddd_7eaa6 : Constant  Value=x_ddd
  Constant_x_l_1ad92 : Constant  Value=x_l
  Constant_x_l_47f7c : Constant  Value=x_l
  Constant_x_l_978b3 : Constant  Value=x_l
  Constant_x_l_a8eea : Constant  Value=x_l
  Constant_x_l_de874 : Constant  Value=x_l
  Constant_x_l_e5275 : Constant  Value=x_l
  Constant_x_qd_749aa : Constant  Value=x_qd
  Constant_x_qd_aa17d : Constant  Value=x_qd
  Constant_x_qd_c9370 : Constant  Value=x_qd
  Constant_x_qdd_95677 : Constant  Value=x_qdd
  Constant_x_qdd_cb821 : Constant  Value=x_qdd
  Constant_x_qdd_f1174 : Constant  Value=x_qdd
  Divide_177cc : Product  Inputs=*/
  Divide_29630 : Product  Inputs=*/
  Divide_58632 : Product  Inputs=*/
  Divide_6dd9a : Product  Inputs=*/
  Divide_7fbed : Product  Inputs=*/
  Divide_8d4e5 : Product  Inputs=*/
  Divide_987fe : Product  Inputs=*/
  Divide_b5d7b : Product  Inputs=*/
  Divide_b64ca : Product  Inputs=*/
  Divide_bf5c3 : Product  Inputs=*/
  MathFunc_sqrt_82adc : Sqrt
  Power_0cdb2 : Math  Operator=pow
  Power_548bb : Math  Operator=pow
  Product_0a284 : Product
  Product_0fcc2 : Product
  Product_254fa : Product
  Product_2833f : Product
  Product_31fae : Product
  Product_52ee6 : Product
  Product_636dc : Product
  Product_67077 : Product
  Product_689e3 : Product
  Product_75569 : Product
  Product_7daab : Product
  Product_8149c : Product
  Product_8b613 : Product
  Product_91c99 : Product
  Product_9def6 : Product
  Product_b005c : Product
  Product_c1142 : Product
  Product_c4180 : Product
  Product_caa5a : Product
  Product_ebdb5 : Product
  Product_edb5d : Product
  Product_f6c6e : Product
  Product_f8892 : Product
  Subtract_3fc92 : Sum  Inputs=+-
  Subtract_45178 : Sum  Inputs=+-
  Subtract_7c679 : Sum  Inputs=+-
  Subtract_7d0d8 : Sum  Inputs=+-
  Subtract_7eb3f : Sum  Inputs=+-
  Subtract_90a92 : Sum  Inputs=+-
  Subtract_a9989 : Sum  Inputs=+-
  Subtract_ab3a9 : Sum  Inputs=+-
  Subtract_d8a6d : Sum  Inputs=+-
  Blockout_d_V_f_SG_D_6_09efe : Outport
  wires:
  Constant_2.0_b4e65/1 -> Product_91c99/1
  Constant_x_qdd_cb821/1 -> Add_3b69d/2
  Constant_-1_be9f7/1 -> Product_caa5a/1
  Constant_x_ddd_7eaa6/1 -> Subtract_a9989/2
  Constant_f0_a4dd1/1 -> Product_f6c6e/2
  Divide_58632/1 -> Subtract_7eb3f/2
  Constant_-1_0eb34/1 -> Product_636dc/1
  Constant_x_qd_c9370/1 -> Add_30c1a/2
  Product_b005c/1 -> Product_0fcc2/1
  Constant_x_l_de874/1 -> Product_636dc/2
  Constant_x_l_47f7c/1 -> Subtract_45178/2
  Constant_-1_c5307/1 -> Product_31fae/1
  Constant_x_l_978b3/1 -> Subtract_7c679/2
  Constant_x_qd_aa17d/1 -> Add_24ee6/2
  Constant_x_dd_d800c/1 -> Subtract_a9989/1
  State_psi_1d_SG_D_6_de2c8/1 -> Product_31fae/2
  Product_636dc/1 -> Add_3b69d/1
  Product_689e3/1 -> Add_df46e/2
  Constant_-1_65e47/1 -> Product_c1142/1
  Constant_x_l_a8eea/1 -> Product_c1142/2
  State_psi_q_SG_D_6_0a3e6/1 -> Product_75569/1
  State_psi_d_SG_D_6_cf70a/1 -> Add_a81f2/2
  Constant_x_qd_749aa/1 -> Subtract_d8a6d/1
  State_w_SG_D_6_e114e/1 -> Product_75569/2
  Constant_x_qdd_95677/1 -> Subtract_d8a6d/2
  Constant_pi_f4b31/1 -> Product_91c99/2
  Constant_x_l_e5275/1 -> Product_caa5a/2
  Product_31fae/1 -> Product_8b613/1
  Constant_R_a_5ff80/1 -> Product_edb5d/1
  Subtract_a9989/1 -> Product_8b613/2
  Constant_2.0_a22ad/1 -> Product_f8892/1
  Constant_-1_8b042/1 -> Product_7daab/1
  Constant_x_dd_4c9ec/1 -> Subtract_7d0d8/1
  Constant_pi_ed0d4/1 -> Product_f8892/2
  Constant_x_l_1ad92/1 -> Subtract_7d0d8/2
  Add_24ee6/1 -> Divide_7fbed/2
  Constant_x_ddd_1897f/1 -> Subtract_45178/1
  State_psi_gq_SG_D_6_73017/1 -> Product_0a284/1
  Add_3b69d/1 -> Product_0a284/2
  Product_c1142/1 -> Add_24ee6/1
  State_psi_kq_SG_D_6_ef584/1 -> Product_67077/1
  Subtract_d8a6d/1 -> Product_67077/2
  Product_91c99/1 -> Product_f6c6e/1
  Constant_-1_713f4/1 -> Product_b005c/1
  Product_caa5a/1 -> Add_30c1a/1
  Product_8b613/1 -> Divide_987fe/1
  Divide_7fbed/1 -> Subtract_3fc92/1
  Subtract_7d0d8/1 -> Divide_987fe/2
  State_psi_fd_SG_D_6_fe54e/1 -> Product_8149c/1
  State_E_fd_SG_D_6_02805/1 -> Product_7daab/2
  Subtract_45178/1 -> Product_8149c/2
  Constant_x_dd_f43c9/1 -> Subtract_7c679/1
  Product_0a284/1 -> Divide_7fbed/1
  Product_67077/1 -> Divide_b64ca/1
  Add_30c1a/1 -> Divide_b64ca/2
  Divide_987fe/1 -> Add_a81f2/1
  Product_8149c/1 -> Divide_58632/1
  Subtract_7c679/1 -> Divide_58632/2
  Divide_b64ca/1 -> Subtract_3fc92/2
  Constant_R_a_3cc7c/1 -> Product_b005c/2
  Add_a81f2/1 -> Subtract_7eb3f/1
  Subtract_3fc92/1 -> Add_cbf81/1
  State_psi_q_SG_D_6_83624/1 -> Add_cbf81/2
  Subtract_7eb3f/1 -> Product_0fcc2/2
  Add_cbf81/1 -> Product_edb5d/2
  State_psi_d_SG_D_6_91b9a/1 -> Product_2833f/1
  State_w_SG_D_6_81790/1 -> Product_2833f/2
  Product_f8892/1 -> Product_254fa/1
  Constant_f0_0dafe/1 -> Product_254fa/2
  Product_0fcc2/1 -> Divide_177cc/1
  Constant_x_ddd_0cd69/1 -> Divide_177cc/2
  Product_75569/1 -> Divide_bf5c3/1
  Product_f6c6e/1 -> Divide_bf5c3/2
  Product_edb5d/1 -> Divide_29630/1
  Constant_x_qdd_f1174/1 -> Divide_29630/2
  Product_2833f/1 -> Divide_6dd9a/1
  Product_254fa/1 -> Divide_6dd9a/2
  Divide_177cc/1 -> Add_a276f/1
  Divide_bf5c3/1 -> Add_a276f/2
  Divide_29630/1 -> Add_6f9c8/1
  Divide_6dd9a/1 -> Add_6f9c8/2
  Add_a276f/1 -> Power_0cdb2/1
  Constant_2.0_0dab5/1 -> Power_0cdb2/2
  Add_6f9c8/1 -> Power_548bb/1
  State_R_f_SG_D_6_28e1c/1 -> Product_ebdb5/2
  Constant_2.0_fe119/1 -> Power_548bb/2
  Product_7daab/1 -> Product_9def6/1
  Constant_K_A_7553d/1 -> Product_9def6/2
  Constant_K_s_866fb/1 -> Product_52ee6/1
  State_Px_3_SG_D_6_bef29/1 -> Product_52ee6/2
  Power_0cdb2/1 -> Add_61ccc/1
  Power_548bb/1 -> Add_61ccc/2
  Product_9def6/1 -> Product_c4180/1
  Constant_K_F_1dd1d/1 -> Product_c4180/2
  Product_52ee6/1 -> Add_f3e8f/1
  Constant_V_ref_ce6f6/1 -> Add_f3e8f/2
  Add_61ccc/1 -> MathFunc_sqrt_82adc/1
  Product_c4180/1 -> Divide_8d4e5/1
  Constant_T_F_aeffc/1 -> Divide_8d4e5/2
  Constant_K_A_32c70/1 -> Product_ebdb5/1
  Add_f3e8f/1 -> Subtract_ab3a9/1
  MathFunc_sqrt_82adc/1 -> Subtract_ab3a9/2
  Divide_8d4e5/1 -> Add_2a290/1
  Product_ebdb5/1 -> Add_2a290/2
  Constant_K_A_59dae/1 -> Product_689e3/1
  Subtract_ab3a9/1 -> Product_689e3/2
  Add_2a290/1 -> Add_df46e/1
  Add_df46e/1 -> Subtract_90a92/1
  State_V_f_SG_D_6_82040/1 -> Subtract_90a92/2
  Subtract_90a92/1 -> Divide_b5d7b/1
  Constant_T_A_98afb/1 -> Divide_b5d7b/2
  Divide_b5d7b/1 -> Blockout_d_V_f_SG_D_6_09efe/1

== system IEEE14_case/SG_D_6/d_psi_1d_SG_D_6_block ==
  note: d_psi_1d_SG_D_6 in case14gfl
      | $-\frac{\psi _{\mathrm{1d},\mathrm{SG},D,6}-\psi _{\mathrm{fd},\mathrm{SG},D,6}+\frac{\left(x_{\mathrm{dd}}-x_{l}\right)\,\left(\frac{\psi _{\mathrm{1d},\mathrm{SG},D,6}\,\left(x_{\mathrm{dd}}-x_{\mathrm{ddd}}\right)}{x_{\mathrm{dd}}-x_{l}}-\psi _{d,\mathrm{SG},D,6}+\frac{\psi _{\mathrm{fd},\mathrm{SG},D,6}\,\left(x_{\mathrm{ddd}}-x_{l}\right)}{x_{\mathrm{dd}}-x_{l}}\right)}{x_{\mathrm{ddd}}}}{T_{\mathrm{ddd}}}$
      | Automatically generated on 2025-10-09 21:33:01 .
  State_psi_1d_SG_D_6_c2ed2 : Inport
  State_psi_fd_SG_D_6_9f319 : Inport  Port=2
  State_psi_1d_SG_D_6_eb113 : Inport  Port=3
  State_psi_d_SG_D_6_4a5c3 : Inport  Port=4
  State_psi_fd_SG_D_6_1aa59 : Inport  Port=5
  Add_071f0 : Sum
  Add_429ad : Sum
  Add_71e10 : Sum
  Constant_-1_134e6 : Constant  Value=-1
  Constant_-1_4d0b7 : Constant  Value=-1
  Constant_T_ddd_f080f : Constant  Value=T_ddd
  Constant_x_dd_3936a : Constant  Value=x_dd
  Constant_x_dd_77d2d : Constant  Value=x_dd
  Constant_x_dd_a3bfe : Constant  Value=x_dd
  Constant_x_dd_d1d84 : Constant  Value=x_dd
  Constant_x_ddd_2429d : Constant  Value=x_ddd
  Constant_x_ddd_4929f : Constant  Value=x_ddd
  Constant_x_ddd_f3cdd : Constant  Value=x_ddd
  Constant_x_l_0f4e0 : Constant  Value=x_l
  Constant_x_l_5dc98 : Constant  Value=x_l
  Constant_x_l_b48ad : Constant  Value=x_l
  Constant_x_l_ee1b3 : Constant  Value=x_l
  Divide_14bdd : Product  Inputs=*/
  Divide_9282b : Product  Inputs=*/
  Divide_bc356 : Product  Inputs=*/
  Divide_cc66e : Product  Inputs=*/
  Product_4d4df : Product
  Product_65cc4 : Product
  Product_78cd2 : Product
  Product_ac8c0 : Product
  Product_e2dae : Product
  Subtract_1400d : Sum  Inputs=+-
  Subtract_21691 : Sum  Inputs=+-
  Subtract_387be : Sum  Inputs=+-
  Subtract_5951a : Sum  Inputs=+-
  Subtract_b5b1c : Sum  Inputs=+-
  Subtract_cbbae : Sum  Inputs=+-
  Blockout_d_psi_1d_SG_D_6_367d1 : Outport
  wires:
  Constant_-1_134e6/1 -> Product_4d4df/1
  State_psi_1d_SG_D_6_eb113/1 -> Product_4d4df/2
  Constant_x_l_5dc98/1 -> Subtract_5951a/2
  Constant_x_ddd_4929f/1 -> Divide_9282b/2
  Product_4d4df/1 -> Product_ac8c0/1
  Constant_x_dd_3936a/1 -> Subtract_387be/1
  Divide_14bdd/1 -> Blockout_d_psi_1d_SG_D_6_367d1/1
  Constant_x_dd_a3bfe/1 -> Subtract_5951a/1
  Product_ac8c0/1 -> Divide_bc356/1
  Constant_x_ddd_f3cdd/1 -> Subtract_387be/2
  Constant_x_l_0f4e0/1 -> Subtract_cbbae/2
  Subtract_387be/1 -> Product_ac8c0/2
  Constant_x_ddd_2429d/1 -> Subtract_cbbae/1
  Subtract_5951a/1 -> Divide_bc356/2
  Divide_9282b/1 -> Add_429ad/2
  Subtract_b5b1c/1 -> Product_e2dae/2
  State_psi_fd_SG_D_6_1aa59/1 -> Product_78cd2/1
  Subtract_cbbae/1 -> Product_78cd2/2
  Constant_x_dd_77d2d/1 -> Subtract_1400d/1
  Add_071f0/1 -> Add_429ad/1
  Constant_x_l_b48ad/1 -> Subtract_1400d/2
  Divide_bc356/1 -> Add_71e10/1
  State_psi_d_SG_D_6_4a5c3/1 -> Add_71e10/2
  Product_78cd2/1 -> Divide_cc66e/1
  Subtract_1400d/1 -> Divide_cc66e/2
  Constant_x_dd_d1d84/1 -> Subtract_21691/1
  Constant_x_l_ee1b3/1 -> Subtract_21691/2
  Add_71e10/1 -> Subtract_b5b1c/1
  Divide_cc66e/1 -> Subtract_b5b1c/2
  Constant_-1_4d0b7/1 -> Product_65cc4/1
  State_psi_1d_SG_D_6_c2ed2/1 -> Product_65cc4/2
  Subtract_21691/1 -> Product_e2dae/1
  Product_65cc4/1 -> Add_071f0/1
  State_psi_fd_SG_D_6_9f319/1 -> Add_071f0/2
  Product_e2dae/1 -> Divide_9282b/1
  Add_429ad/1 -> Divide_14bdd/1
  Constant_T_ddd_f080f/1 -> Divide_14bdd/2

== system IEEE14_case/SG_D_6/d_psi_d_SG_D_6_block ==
  note: d_psi_d_SG_D_6 in case14gfl
      | $2\,\pi \,f_{0}\,\left(v_{d,\mathrm{SG},D,6}\,\sin\left(\theta _{\mathrm{SG},D,6}\right)-v_{q,\mathrm{SG},D,6}\,\cos\left(\theta _{\mathrm{SG},D,6}\right)+\frac{R_{a}\,\left(\frac{\psi _{\mathrm{1d},\mathrm{SG},D,6}\,\left(x_{\mathrm{dd}}-x_{\mathrm{ddd}}\right)}{x_{\mathrm{dd}}-x_{l}}-\psi _{d,\mathrm{SG},D,6}+\frac{\psi _{\mathrm{fd},\mathrm{SG},D,6}\,\left(x_{\mathrm{ddd}}-x_{l}\right)}{x_{\mathrm{dd}}-x_{l}}\right)}{x_{\mathrm{ddd}}}+\frac{\psi _{q,\mathrm{SG},D,6}\,w_{\mathrm{SG},D,6}}{2\,f_{0}\,\pi }\right)$
      | Automatically generated on 2025-10-09 21:32:50 .
  State_psi_1d_SG_D_6_101db : Inport
  State_psi_d_SG_D_6_c802b : Inport  Port=2
  State_psi_fd_SG_D_6_200cb : Inport  Port=3
  Input_v_d_SG_D_6_af95d : Inport  Port=4
  State_theta_SG_D_6_4b87e : Inport  Port=5
  Input_v_q_SG_D_6_c8c76 : Inport  Port=6
  State_theta_SG_D_6_acea8 : Inport  Port=7
  State_psi_q_SG_D_6_65dc8 : Inport  Port=8
  State_w_SG_D_6_f3bca : Inport  Port=9
  Add_13b99 : Sum
  Add_b594c : Sum
  Constant_-1_a1d11 : Constant  Value=-1
  Constant_-2.0_24bda : Constant  Value=-2.0
  Constant_2.0_a6ee8 : Constant  Value=2.0
  Constant_R_a_1bfbd : Constant  Value=R_a
  Constant_f0_02510 : Constant  Value=f0
  Constant_f0_41e53 : Constant  Value=f0
  Constant_pi_9a179 : Constant  Value=pi
  Constant_pi_b7e67 : Constant  Value=pi
  Constant_x_dd_0aa88 : Constant  Value=x_dd
  Constant_x_dd_5973f : Constant  Value=x_dd
  Constant_x_dd_7a461 : Constant  Value=x_dd
  Constant_x_ddd_1d29b : Constant  Value=x_ddd
  Constant_x_ddd_a5aef : Constant  Value=x_ddd
  Constant_x_ddd_c5766 : Constant  Value=x_ddd
  Constant_x_l_293e3 : Constant  Value=x_l
  Constant_x_l_4e570 : Constant  Value=x_l
  Constant_x_l_eb323 : Constant  Value=x_l
  Divide_17521 : Product  Inputs=*/
  Divide_4692a : Product  Inputs=*/
  Divide_50768 : Product  Inputs=*/
  Divide_969f4 : Product  Inputs=*/
  MathFunc_cos_5cafd : Trigonometry  Operator=cos
  MathFunc_sin_6a9f1 : Trigonometry
  Product_04e3f : Product
  Product_08fa6 : Product
  Product_0a90f : Product
  Product_17ee6 : Product
  Product_217c7 : Product
  Product_440e6 : Product
  Product_682e0 : Product
  Product_80d76 : Product
  Product_82dd1 : Product
  Product_8f6f9 : Product
  Product_9094a : Product
  Product_ca3e3 : Product
  Subtract_105fc : Sum  Inputs=+-
  Subtract_3e430 : Sum  Inputs=+-
  Subtract_49732 : Sum  Inputs=+-
  Subtract_4ee68 : Sum  Inputs=+-
  Subtract_7aaf2 : Sum  Inputs=+-
  Subtract_8657f : Sum  Inputs=+-
  Subtract_ce1bf : Sum  Inputs=+-
  Blockout_d_psi_d_SG_D_6_3b081 : Outport
  wires:
  Constant_-1_a1d11/1 -> Product_80d76/1
  Product_9094a/1 -> Product_440e6/1
  Subtract_7aaf2/1 -> Product_ca3e3/2
  State_theta_SG_D_6_4b87e/1 -> MathFunc_sin_6a9f1/1
  State_psi_1d_SG_D_6_101db/1 -> Product_80d76/2
  Constant_2.0_a6ee8/1 -> Product_9094a/1
  Constant_x_dd_7a461/1 -> Subtract_7aaf2/1
  Constant_pi_b7e67/1 -> Product_9094a/2
  Constant_x_ddd_1d29b/1 -> Subtract_7aaf2/2
  Product_80d76/1 -> Product_ca3e3/1
  Constant_x_dd_5973f/1 -> Subtract_105fc/1
  Constant_x_l_293e3/1 -> Subtract_105fc/2
  Constant_x_ddd_c5766/1 -> Subtract_ce1bf/1
  Constant_x_l_eb323/1 -> Subtract_ce1bf/2
  State_psi_q_SG_D_6_65dc8/1 -> Product_0a90f/1
  Product_ca3e3/1 -> Divide_969f4/1
  Subtract_105fc/1 -> Divide_969f4/2
  State_psi_fd_SG_D_6_200cb/1 -> Product_08fa6/1
  Constant_R_a_1bfbd/1 -> Product_82dd1/1
  Subtract_ce1bf/1 -> Product_08fa6/2
  Constant_-2.0_24bda/1 -> Product_682e0/1
  Constant_x_dd_0aa88/1 -> Subtract_49732/1
  Constant_x_l_4e570/1 -> Subtract_49732/2
  Divide_969f4/1 -> Add_b594c/1
  State_psi_d_SG_D_6_c802b/1 -> Add_b594c/2
  Product_08fa6/1 -> Divide_17521/1
  Subtract_49732/1 -> Divide_17521/2
  Add_b594c/1 -> Subtract_4ee68/1
  Divide_17521/1 -> Subtract_4ee68/2
  Subtract_4ee68/1 -> Product_82dd1/2
  State_theta_SG_D_6_acea8/1 -> MathFunc_cos_5cafd/1
  Product_82dd1/1 -> Divide_4692a/1
  Product_682e0/1 -> Product_04e3f/1
  Constant_x_ddd_a5aef/1 -> Divide_4692a/2
  Input_v_d_SG_D_6_af95d/1 -> Product_8f6f9/1
  Divide_4692a/1 -> Subtract_3e430/1
  MathFunc_sin_6a9f1/1 -> Product_8f6f9/2
  Product_8f6f9/1 -> Subtract_3e430/2
  Input_v_q_SG_D_6_c8c76/1 -> Product_17ee6/1
  MathFunc_cos_5cafd/1 -> Product_17ee6/2
  State_w_SG_D_6_f3bca/1 -> Product_0a90f/2
  Constant_f0_02510/1 -> Product_440e6/2
  Constant_pi_9a179/1 -> Product_682e0/2
  Subtract_3e430/1 -> Add_13b99/1
  Product_17ee6/1 -> Add_13b99/2
  Product_0a90f/1 -> Divide_50768/1
  Product_440e6/1 -> Divide_50768/2
  Constant_f0_41e53/1 -> Product_04e3f/2
  Add_13b99/1 -> Subtract_8657f/1
  Divide_50768/1 -> Subtract_8657f/2
  Product_04e3f/1 -> Product_217c7/1
  Subtract_8657f/1 -> Product_217c7/2
  Product_217c7/1 -> Blockout_d_psi_d_SG_D_6_3b081/1
